simulink model "FuzzyPIDtesting"  (R2016a)
settings: Solver=VariableStepAuto  StartTime=0.0  StopTime=10.0  RelTol=1e-3
values from neighbouring files (symbols this model uses):
  Bm = 0.002953    [April2code.mat]    (also in April6code.mat)
  Jm = 0.02215    [April2code.mat]    (also in April6code.mat)
  Kb = 1.28    [April2code.mat]    (also in April6code.mat)
  Kt = 1.28    [April2code.mat]    (also in April6code.mat)
  La = 0.1215    [April2code.mat]    (also in April6code.mat)
  Ra = 11.2    [April2code.mat]    (also in April6code.mat)
libraries: simulink x1
settings Model: Creator=Dheeraj Singh  LastModifiedBy=Dheeraj Singh

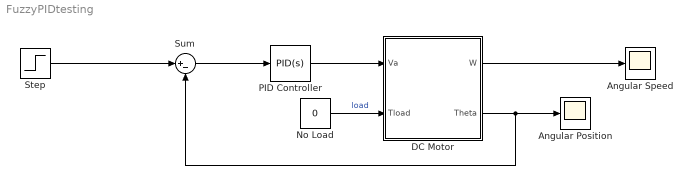
== system FuzzyPIDtesting ==
  Angular Position : Scope
  Angular Speed : Scope
  DC Motor : Subsystem
  No Load : Constant  Value=0
  PID Controller : simulink/Continuous/PID Controller  Controller=PID  TimeDomain=Continuous-time  SampleTime=-1  IntegratorMethod=Forward Euler  FilterMethod=Forward Euler  Form=Parallel  UseFilter=on  ControllerParametersSource=internal  P=15  I=0.01  D=3  N=100  InitialConditionSource=internal  InitialConditionForIntegrator=0  InitialConditionForFilter=0  ExternalReset=none  LimitOutput=off  UpperSaturationLimit=inf  LowerSaturationLimit=-inf  LinearizeAsGain=on  AntiWindupMode=none  Kb=1  TrackingMode=off  Kt=1  PParamMin=[]  PParamMax=[]  IParamMin=[]  IParamMax=[]  DParamMin=[]  DParamMax=[]  NParamMin=[]  NParamMax=[]  KbParamMin=[]  KbParamMax=[]  KtParamMin=[]  KtParamMax=[]  POutMin=[]  POutMax=[]  IOutMin=[]  IOutMax=[]  DOutMin=[]  DOutMax=[]  NOutMin=[]  NOutMax=[]  KbOutMin=[]  KbOutMax=[]  KtOutMin=[]  KtOutMax=[]  IntegratorOutMin=[]  IntegratorOutMax=[]  FilterOutMin=[]  FilterOutMax=[]  SumOutMin=[]  SumOutMax=[]  SumI1OutMin=[]  SumI1OutMax=[]  SumI2OutMin=[]  SumI2OutMax=[]  SumI3OutMin=[]  SumI3OutMax=[]  SumDOutMin=[]  SumDOutMax=[]  SaturationOutMin=[]  SaturationOutMax=[]  IntegratorContinuousStateAttributes=''  IntegratorStateMustResolveToSignalObject=off  IntegratorRTWStateStorageClass=Auto  FilterContinuousStateAttributes=''  FilterStateMustResolveToSignalObject=off  FilterRTWStateStorageClass=Auto  DifferentiatorICPrevScaledInput=0  DifferentiatorOutMin=[]  DifferentiatorOutMax=[]
  Step : Step  SampleTime=0
  Sum : Sum  Inputs=|+-
  wires:
  PID Controller/1 -> DC Motor/1(Va)
  No Load/1 -> DC Motor/2(Tload)  "load"
  DC Motor/2(Theta) -> Sum/2, Angular Position/1
  Step/1 -> Sum/1
  Sum/1 -> PID Controller/1
  DC Motor/1(W) -> Angular Speed/1

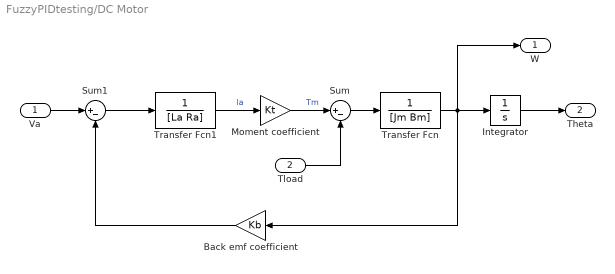
== system FuzzyPIDtesting/DC Motor ==
  Va : Inport
  Tload : Inport  Port=2
  Back emf coefficient : Gain  Gain=Kb
  Integrator : Integrator
  Moment coefficient : Gain  Gain=Kt
  Sum : Sum  Inputs=|+-
  Sum1 : Sum  Inputs=|+-
  Transfer Fcn : TransferFcn  Denominator=[Jm Bm]
  Transfer Fcn1 : TransferFcn  Denominator=[La Ra]
  W : Outport
  Theta : Outport  Port=2
  wires:
  Transfer Fcn1/1 -> Moment coefficient/1  "la"
  Sum/1 -> Transfer Fcn/1
  Va/1 -> Sum1/1
  Moment coefficient/1 -> Sum/1  "Tm"
  Transfer Fcn/1 -> W/1, Back emf coefficient/1, Integrator/1
  Integrator/1 -> Theta/1
  Tload/1 -> Sum/2
  Sum1/1 -> Transfer Fcn1/1
  Back emf coefficient/1 -> Sum1/2
